simulink model "Gesamtsystem"  (R2018b)
settings: Solver=FixedStepDiscrete  StartTime=0.0  StopTime=1  RelTol=1e-3  EnableMultiTasking=on
libraries: c2833xlib x12, commutil2 x12, c280xlib x9, powerlib_extras x2, simulink x1, c2000lib x1, dspstat3 x1
(part 2 of 3)

== system Gesamtsystem/Subsystem/Subsystem2 ==
  In1 : Inport
  In2 : Inport  Port=2
  Drehrichtungsvorgabe für einen Motor1 : c2833xlib/Digital Output  GPIO_Number=GPIO16~GPIO23  GPIO_Bit0=on  GPIO_BIT0_Toggle=off  GPIO_Bit1=off  GPIO_BIT1_Toggle=off  GPIO_Bit2=off  GPIO_BIT2_Toggle=off  GPIO_Bit3=off  GPIO_BIT3_Toggle=off  GPIO_Bit4=off  GPIO_BIT4_Toggle=off  GPIO_Bit5=off  GPIO_BIT5_Toggle=off  GPIO_Bit6=off  GPIO_BIT6_Toggle=off  GPIO_Bit7=off  GPIO_BIT7_Toggle=off
      settings: SourceProductName=Embedded Coder Support Package for Texas Instruments C2000 Processors  SourceProductBaseCode=TIC2000
  PWM Vorgabe für einen Motor 1 : c280xlib/ePWM  checkMode=off  useModule=ePWM6  periodUnits=Clock cycles  timerSource=Specify via dialog  timerPeriod_clk=64000  timerPeriod_sec=0.0001  tbshadow=Counter equals to zero  countingMode=Up  phaseActiveEnable=Disable  phaseDirection=Count down after sync  phaseActive=0  synchronizationEnable=off  synchronizationOption=Disable  clockPrescale=1  HSclockPrescale=1  ePWMxAStatus=off  CMPAUnits=Clock cycles  CMPASource=Specify via dialog  CMPAValue_per=50  CMPAValue_clk=32000  enCMPAshadow=Counter equals to zero  ePWMxAactionLogic1=Do nothing  ePWMxAactionLogic2=Clear  ePWMxAactionLogic3=Set  ePWMxAactionLogic4=Do nothing  ePWMxAactionLogic5=Do nothing  ePWMxAactionLogic6=Do nothing  ePWMxALoadMode=Load on counter equals to zero (CTR=Zero)  ePWMxACSFenable=off  ePWMxACSFvalue=Forcing disable  ePWMxASFreload=Zero  enHRPWM=off  HRPWM_LoadMode=Counter equals to zero (CTR=ZERO)  HRPWM_CTLMode=Phase control mode  HRPWM_EDGMode=Both edge  enSFO=on  ePWMxBStatus=on  CMPBUnits=Percentages  CMPBSource=Input port  CMPBValue_per=0  CMPBValue_clk=32000  enCMPBshadow=Counter equals to zero  ePWMxBactionLogic1=Do nothing  ePWMxBactionLogic2=Set  ePWMxBactionLogic3=Do nothing  ePWMxBactionLogic4=Do nothing  ePWMxBactionLogic5=Clear  ePWMxBactionLogic6=Do nothing  ePWMxBLoadMode=Load on counter equals to zero (CTR=Zero)  ePWMxBCSFenable=off  ePWMxBCSFvalue=Forcing disable  ePWMxBSFreload=Zero  enableDBePWMxA=off  enableDBePWMxB=off  DBpolarity=Active high (AH)  DBedgeDelay=Positive  DBSource_ePWMxA=ePWMxA  DBSource_ePWMxB=ePWMxA  DBperiodSource=Specify via dialog  REDperiod=0  FEDperiod=0  adcstartModuleA=off  adcrequestEventA=First event  adcstartEventA=Counter equals to zero (CTR=Zero)  adcstartModuleB=off  adcrequestEventB=First event  adcstartEventB=Counter equals to zero (CTR=Zero)  intEn=off  intPrd=First event  intSel=Counter equals to zero (CTR=Zero)  chopperEnable=off  chopperFrequency=1  chopperFirstwidth=1  chopperDuty=12.5%  tripZonesource=Specify via dialog  tzselOSHT1=off  tzselOSHT2=off  tzselOSHT3=off  tzselOSHT4=off  tzselOSHT5=off  tzselOSHT6=off  tzselCBC1=off  tzselCBC2=off  tzselCBC3=off  tzselCBC4=off  tzselCBC5=off  tzselCBC6=off  enTzOstIntr=off  enTzCbcIntr=off  ePWMxAforced=No action  ePWMxBforced=No action  timerPeriod=-1  ePWMxAValue=0  ePWMxBValue=0  tripZoneoption=One-shot trip (OSHT)
      settings: SourceProductName=Embedded Coder Support Package for Texas Instruments C2000 Processors  SourceProductBaseCode=TIC2000
  wires:
  In2/1 -> Drehrichtungsvorgabe für einen Motor1/1
  In1/1 -> PWM Vorgabe für einen Motor 1/1

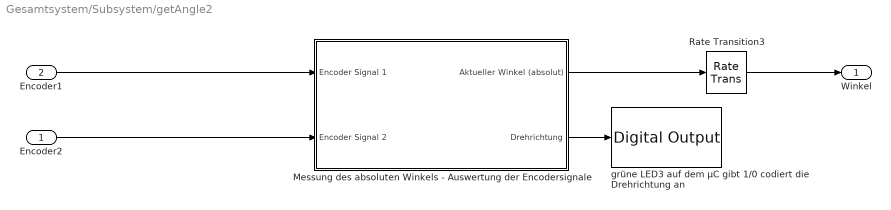
== system Gesamtsystem/Subsystem/getAngle2 ==
  Encoder2 : Inport
  Encoder1 : Inport  Port=2
  Messung des absoluten Winkels - Auswertung der Encodersignale : Subsystem
  Rate Transition3 : RateTransition  OutPortSampleTime=0.01
  grüne LED3 auf dem µC gibt 1/0 codiert die Drehrichtung an : c2833xlib/Digital Output  GPIO_Number=GPIO32~GPIO39  GPIO_Bit0=off  GPIO_BIT0_Toggle=off  GPIO_Bit1=off  GPIO_BIT1_Toggle=off  GPIO_Bit2=on  GPIO_BIT2_Toggle=off  GPIO_Bit3=off  GPIO_BIT3_Toggle=off  GPIO_Bit4=off  GPIO_BIT4_Toggle=off  GPIO_Bit5=off  GPIO_BIT5_Toggle=off  GPIO_Bit6=off  GPIO_BIT6_Toggle=off  GPIO_Bit7=off  GPIO_BIT7_Toggle=off
      settings: SourceProductName=Embedded Coder Support Package for Texas Instruments C2000 Processors  SourceProductBaseCode=TIC2000
  Winkel : Outport
  wires:
  Encoder1/1 -> Messung des absoluten Winkels - Auswertung der Encodersignale/1(Encoder Signal 1)
  Messung des absoluten Winkels - Auswertung der Encodersignale/2(Drehrichtung) -> grüne LED3 auf dem µC gibt 1/0 codiert die Drehrichtung an/1
  Messung des absoluten Winkels - Auswertung der Encodersignale/1(Aktueller Winkel (absolut)) -> Rate Transition3/1
  Encoder2/1 -> Messung des absoluten Winkels - Auswertung der Encodersignale/2(Encoder Signal 2)
  Rate Transition3/1 -> Winkel/1

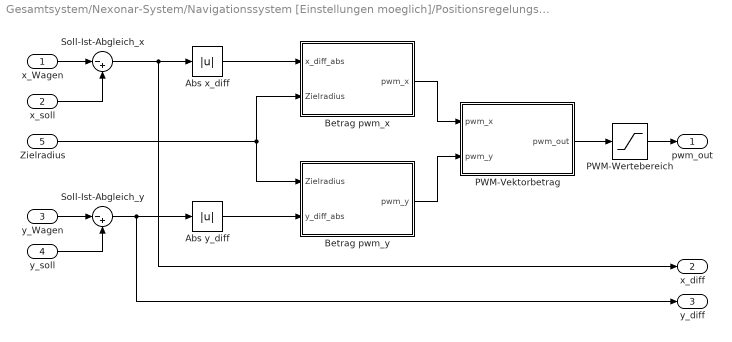
== system Gesamtsystem/Nexonar-System/Navigationssystem [Einstellungen moeglich]/Positionsregelungssystem (Soll-Ist-Abgleich & PWM-Auswertung) ==
  x_Wagen : Inport
  x_soll : Inport  Port=2
  y_Wagen : Inport  Port=3
  y_soll : Inport  Port=4
  Zielradius : Inport  Port=5
  Abs x_diff : Abs  SampleTime=0.01
  Abs y_diff : Abs  SampleTime=0.01
  Betrag pwm_x : MATLAB Function  TreatAsAtomicUnit=on  SystemSampleTime=0.01
  Betrag pwm_y : MATLAB Function  TreatAsAtomicUnit=on  SystemSampleTime=0.01
  PWM-Vektorbetrag : MATLAB Function  TreatAsAtomicUnit=on
  PWM-Wertebereich : Saturate  UpperLimit=100  LowerLimit=0
  Soll-Ist-Abgleich_x : Sum  Inputs=|-+  SampleTime=0.01
  Soll-Ist-Abgleich_y : Sum  Inputs=|-+  AccumDataTypeStr=double  SampleTime=0.01
  pwm_out : Outport
  x_diff : Outport  Port=2
  y_diff : Outport  Port=3
  wires:
  Soll-Ist-Abgleich_x/1 -> x_diff/1, Abs x_diff/1
  Abs x_diff/1 -> Betrag pwm_x/1(x_diff_abs)
  x_soll/1 -> Soll-Ist-Abgleich_x/2
  x_Wagen/1 -> Soll-Ist-Abgleich_x/1
  y_Wagen/1 -> Soll-Ist-Abgleich_y/1
  y_soll/1 -> Soll-Ist-Abgleich_y/2
  Soll-Ist-Abgleich_y/1 -> Abs y_diff/1, y_diff/1
  Abs y_diff/1 -> Betrag pwm_y/2(y_diff_abs)
  PWM-Wertebereich/1 -> pwm_out/1
  PWM-Vektorbetrag/1(pwm_out) -> PWM-Wertebereich/1
  Betrag pwm_x/1(pwm_x) -> PWM-Vektorbetrag/1(pwm_x)
  Betrag pwm_y/1(pwm_y) -> PWM-Vektorbetrag/2(pwm_y)
  Zielradius/1 -> Betrag pwm_y/1(Zielradius), Betrag pwm_x/2(Zielradius)

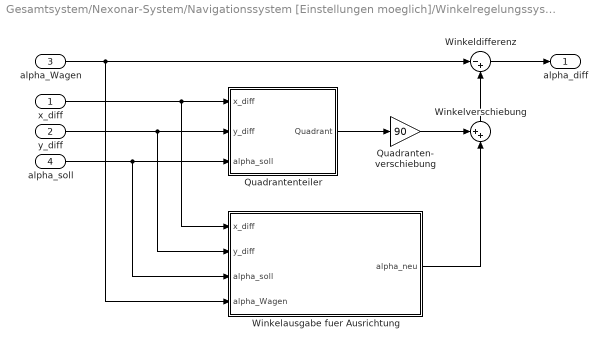
== system Gesamtsystem/Nexonar-System/Navigationssystem [Einstellungen moeglich]/Winkelregelungssystem (Soll-Ist-Abgleich & Ausrichtungsauswertung) ==
  x_diff : Inport
  y_diff : Inport  Port=2
  alpha_Wagen : Inport  Port=3
  alpha_soll : Inport  Port=4
  Quadranten- verschiebung : Gain  Gain=90
  Quadrantenteiler : Stateflow chart  TreatAsAtomicUnit=on
  Winkelausgabe fuer Ausrichtung : Stateflow chart  TreatAsAtomicUnit=on
  Winkeldifferenz : Sum  Inputs=|-+
  Winkelverschiebung : Sum  Inputs=++|
  alpha_diff : Outport
  wires:
  alpha_Wagen/1 -> Winkelausgabe fuer Ausrichtung/4(alpha_Wagen), Winkeldifferenz/1
  y_diff/1 -> Winkelausgabe fuer Ausrichtung/2(y_diff), Quadrantenteiler/2(y_diff)
  Winkelausgabe fuer Ausrichtung/1(alpha_neu) -> Winkelverschiebung/2
  Winkelverschiebung/1 -> Winkeldifferenz/2
  x_diff/1 -> Winkelausgabe fuer Ausrichtung/1(x_diff), Quadrantenteiler/1(x_diff)
  Quadrantenteiler/1(Quadrant) -> Quadranten- verschiebung/1
  Winkeldifferenz/1 -> alpha_diff/1
  Quadranten- verschiebung/1 -> Winkelverschiebung/1
  alpha_soll/1 -> Winkelausgabe fuer Ausrichtung/3(alpha_soll), Quadrantenteiler/3(alpha_soll)

== system Gesamtsystem/Nexonar-System/Nexonar-Positionsbestimmung/I2C Reset (behebt Stabilitätsprobleme der I2C-Verbindung) ==
  I2C Reinitialisierung : Subsystem  TreatAsAtomicUnit=on
  I2C Reset : Subsystem  TreatAsAtomicUnit=on
  Pulse Generator : DiscretePulseGenerator  Period=250  SampleTime=0.01
  wires:
  Pulse Generator/1 -> I2C Reinitialisierung/Trigger, I2C Reset/Trigger

== system Gesamtsystem/Nexonar-System/Nexonar-Positionsbestimmung/Triggered Subsystem ==
  Trigger : TriggerPort  TriggerType=function-call  VariantControl=(inherit)
  Delay : Delay  DelayLength=1  InitialCondition=0
  I2C Receive : c280xlib/I2C Receive  selectModule=I2C_A  addrFormat=7-Bit addressing  saSource=Specify via dialog  SAR=80  bitCount=8  dataLength=10  initValue=0  NACK=on  STP=off  STR=on  sampleTime=-1  dataType=uint8
      settings: SourceProductName=Embedded Coder Support Package for Texas Instruments C2000 Processors  SourceProductBaseCode=TIC2000
  Terminator : Terminator
  Vector Concatenate : Concatenate
  I2C_Read_Data : Outport
  wires:
  I2C Receive/2 -> Terminator/1
  I2C Receive/1 -> Vector Concatenate/2, Delay/1
  Delay/1 -> Vector Concatenate/1
  Vector Concatenate/1 -> I2C_Read_Data/1

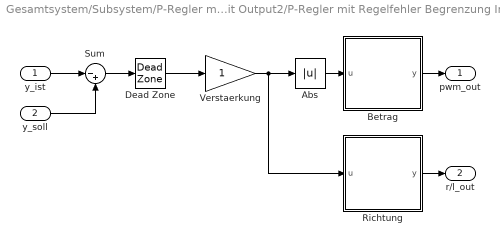
== system Gesamtsystem/Subsystem/P-Regler mit Output2/P-Regler mit Regelfehler Begrenzung Initial: k = 0.1, limiit = +//- 100 Sampletime 0.01 ==
  y_ist : Inport
  y_soll : Inport  Port=2
  Abs : Abs  SampleTime=0.01
  Betrag : MATLAB Function  TreatAsAtomicUnit=on  SystemSampleTime=0.01
  Dead Zone : DeadZone  SampleTime=0.01  SaturateOnIntegerOverflow=on
  Richtung : MATLAB Function  TreatAsAtomicUnit=on  SystemSampleTime=0.01
  Sum : Sum  Inputs=|-+  SampleTime=0.01
  Verstaerkung : Gain  SampleTime=0.01
  pwm_out : Outport
  r/l_out : Outport  Port=2
  wires:
  Betrag/1(y) -> pwm_out/1
  Sum/1 -> Dead Zone/1
  Verstaerkung/1 -> Abs/1, Richtung/1(u)
  Dead Zone/1 -> Verstaerkung/1
  Abs/1 -> Betrag/1(u)
  y_soll/1 -> Sum/2
  Richtung/1(y) -> r/l_out/1
  y_ist/1 -> Sum/1

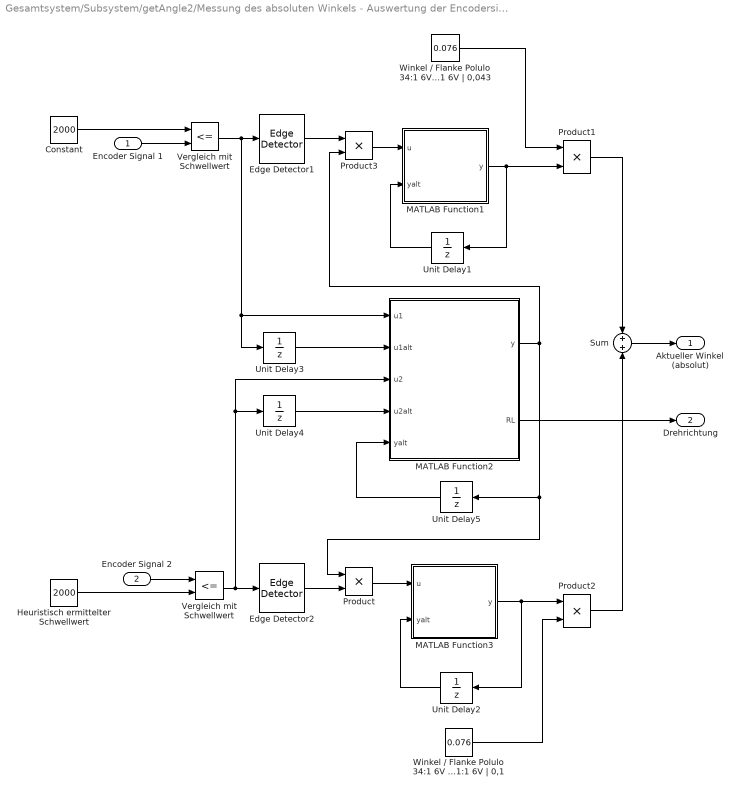
== system Gesamtsystem/Subsystem/getAngle2/Messung des absoluten Winkels - Auswertung der Encodersignale ==
  Encoder Signal 1 : Inport
  Encoder Signal 2 : Inport  Port=2
  Constant : Constant  Value=2000
  Edge Detector1 : powerlib_extras/Control  Blocks/Edge Detector  model=Either  ic=0
  Edge Detector2 : powerlib_extras/Control  Blocks/Edge Detector  model=Either  ic=0
  Heuristisch ermittelter Schwellwert : Constant  Value=2000
  MATLAB Function1 : MATLAB Function  TreatAsAtomicUnit=on
  MATLAB Function2 : MATLAB Function  TreatAsAtomicUnit=on
  MATLAB Function3 : MATLAB Function  TreatAsAtomicUnit=on
  Product{,1..3} (4 alike) : Product  RndMeth=Zero
  Sum : Sum  Inputs=+|+
  Unit Delay{1..5} (5 alike) : UnitDelay  SampleTime=-1
  Vergleich mit Schwellwert : RelationalOperator  Operator=<=  OutDataTypeStr=boolean  RndMeth=Nearest
  Vergleich mit Schwellwert : RelationalOperator  Operator=<=  OutDataTypeStr=boolean  RndMeth=Nearest
  Winkel / Flanke Polulo 34:1 6V | 0,22 Polulo 74:1 6V | 0,1 Polulo 98:1 6V | 0,076 Polulo 171:1 6V | 0,043 : Constant  Value=0.076
  Winkel / Flanke Polulo 34:1 6V | 0,22 Polulo 74:1 6V | 0,1 Polulo 98:1 6V | 0,076 Polulo 171:1 6V | 0,1 : Constant  Value=0.076
  Aktueller Winkel (absolut) : Outport
  Drehrichtung : Outport  Port=2
  wires:
  Vergleich mit Schwellwert/1 -> Unit Delay4/1, MATLAB Function2/3(u2), Edge Detector2/1
  Sum/1 -> Aktueller Winkel (absolut)/1
  Vergleich mit Schwellwert/1 -> Edge Detector1/1, Unit Delay3/1, MATLAB Function2/1(u1)
  Heuristisch ermittelter Schwellwert/1 -> Vergleich mit Schwellwert/2
  Unit Delay2/1 -> MATLAB Function3/2(yalt)
  Encoder Signal 1/1 -> Vergleich mit Schwellwert/2
  MATLAB Function3/1(y) -> Unit Delay2/1, Product2/1
  Product1/1 -> Sum/1
  Constant/1 -> Vergleich mit Schwellwert/1
  Encoder Signal 2/1 -> Vergleich mit Schwellwert/1
  Product2/1 -> Sum/2
  Unit Delay1/1 -> MATLAB Function1/2(yalt)
  MATLAB Function1/1(y) -> Product1/2, Unit Delay1/1
  Winkel / Flanke Polulo 34:1 6V | 0,22 Polulo 74:1 6V | 0,1 Polulo 98:1 6V | 0,076 Polulo 171:1 6V | 0,043/1 -> Product1/1
  Product3/1 -> MATLAB Function1/1(u)
  Product/1 -> MATLAB Function3/1(u)
  Edge Detector1/1 -> Product3/1
  Unit Delay3/1 -> MATLAB Function2/2(u1alt)
  Unit Delay4/1 -> MATLAB Function2/4(u2alt)
  Edge Detector2/1 -> Product/2
  MATLAB Function2/1(y) -> Product/1, Unit Delay5/1, Product3/2
  Winkel / Flanke Polulo 34:1 6V | 0,22 Polulo 74:1 6V | 0,1 Polulo 98:1 6V | 0,076 Polulo 171:1 6V | 0,1/1 -> Product2/2
  MATLAB Function2/2(RL) -> Drehrichtung/1
  Unit Delay5/1 -> MATLAB Function2/5(yalt)

== system Gesamtsystem/Nexonar-System/Nexonar-Positionsbestimmung/I2C Reset (behebt Stabilitätsprobleme der I2C-Verbindung)/I2C Reinitialisierung ==
  Trigger : TriggerPort  TriggerType=falling  VariantControl=(inherit)
  I2C Reinitialisierung : MATLAB Function  TreatAsAtomicUnit=on

== system Gesamtsystem/Nexonar-System/Nexonar-Positionsbestimmung/I2C Reset (behebt Stabilitätsprobleme der I2C-Verbindung)/I2C Reset ==
  Trigger : TriggerPort  VariantControl=(inherit)
  I2C Reset : MATLAB Function  TreatAsAtomicUnit=on

== stateflow chart Gesamtsystem/Nexonar-System/Nexonar-Positionsbestimmung/Chart1 ==
  state Daten_einlesen
  state x0
  state x1_1
    entry: int16z_bin[0] = int8z_1[0];
    int16z_bin[1] = int8z_1[1];
    int16z_bin[2] = int8z_1[2];
    int16z_bin[3] = int8z_1[3];
    int16z_bin[4] = int8z_1[4];
    int16z_bin[5] = int8z_1[5]
    int16z_bin[6] = int8z_1[6];
    int16z_bin[7] = int8z_1[7];
    int16z_bin[8] = int8z_2[0];
    int16z_bin[9] = int8z_2[1];
    int16z_bin[10] = int8z_2[2];
    int16z_bin[11] = int8z_2[3];
    int16z_bin[12] = int8z_2[4];
    int16z_bin[13] = int8z_2[5]
    int16z_bin[14] = int8z_2[6];
    int16z_bin[15] = int8z_2[7];
  x0 -> Daten_einlesen
  (default) -> x0
  Daten_einlesen -> x1_1
  x1_1 -> Daten_einlesen
  data: int8z_1 input size=8; int8z_2 input size=8; int16z_bin output size=16 =0

== matlab function Gesamtsystem/Nexonar-System/Navigationssystem [Einstellungen moeglich]/Positionsregelungssystem (Soll-Ist-Abgleich & PWM-Auswertung)/PWM-Vektorbetrag ==
  data: pwm_x input; pwm_out output; pwm_y input
function pwm_out = fcn(pwm_x, pwm_y)

pwm_out = round(sqrt(pwm_x * pwm_x + pwm_y * pwm_y));

== stateflow chart Gesamtsystem/Add-Ons-Ansteuerung [Einstellungen moeglich] Achtung! Einige Einstellungswerte haengen von den Werten im Nexonar-System ab./Beendigung-System [Einstellungen moeglich]/Beendigung-Ansteuerung ==
  state Start_Warten
  state Aus_Zustand
    entry:
    aus_an = 0;
  state Anschalten
    entry:
    aus_an = 1;
  (default) -> Start_Warten
  Start_Warten -> Aus_Zustand
  Aus_Zustand -> Anschalten [order 1] : [Shutdown == 1]
  Aus_Zustand -> Anschalten [order 2] : [Fahrzeug_Motoren(1) == 0 && Fahrzeug_Motoren(2) == 0 ...
      | && Fahrzeug_Motoren(3) == Fahrzeug_Motoren(4)]
  data: aus_an output; Fahrzeug_Motoren input; Shutdown input

== matlab function Gesamtsystem/Nexonar-System/Konvertierung Nexonar -> Fahrzeug Folgende Werte koennen für Nexonar eingestellt werden: - r_Versatz_Nexo: Radialer Versatz des Nexonars zur Rotationsachse des Fahrzeugs - phi_Versatz_Nexo: Winkelversatz des Nexonars gegenüber der x-Achse (Mittelpunkt: Rotationspunkt des Fahrzeugs) - psi_Offset_Nexo: Winkelversatz des Nexonars gegenüber der x-Achse (Mittelpunkt: Nexonar-Empfangstelle) ==
  data: x_ist input; x_Wagen output; y_ist input; alpha_ist input; y_Wagen output; alpha_Wagen output
function [x_Wagen, y_Wagen, alpha_Wagen] = fcn(x_ist, y_ist, alpha_ist)

r_Versatz_Nexo = 2.5; % in mm
phi_Versatz_Nexo = 30; % in °
psi_Offset_Nexo = 15; % in 


alpha_Wagen = alpha_ist - psi_Offset_Nexo;
x_Wagen = x_ist - round(r_Versatz_Nexo * cos((phi_Versatz_Nexo+alpha_Wagen)*2*pi/360));
y_Wagen = y_ist - round(r_Versatz_Nexo * sin((phi_Versatz_Nexo+alpha_Wagen)*2*pi/360));

== stateflow chart Gesamtsystem/Nexonar-System/Fahrablaufsteuerung [Init: Zielradius = 10mm] Gang = 0: vorwaerts Gang = 1: rueckwaerts Folgende Werte fuer den Ablauf sind einstellbar: - Zielkoordinatenwerte - Gangwert ==
  state Parken
    state Parken_1
      entry:
      x_soll = 1420;
      y_soll = -50;
      alpha_soll = -1;
    state Wechsel_1
      entry:
      Counter = Counter + 1;
    state Parken_2
      entry:
      x_soll = 1620;
      y_soll = -135;
      alpha_soll = -1;
    state Wechsel_2
      entry:
      Counter = Counter + 1;
    state Parken_3
      entry:
      x_soll = 1640;
      y_soll = -131;
      alpha_soll = -1;
    state Wechsel_3
      entry:
      Counter = Counter + 1;
    (default) -> Parken_1 : {Counter = 0}
    Parken_1 -> Parken.Wechsel_1 : [abs(x_soll - x_Wagen) <= Zielradius && abs(y_soll - y_Wagen) <= Zielradius]
    Parken.Wechsel_1 -> Parken_2
    Parken_2 -> Parken.Wechsel_2 : [abs(x_soll - x_Wagen) <= Zielradius && abs(y_soll - y_Wagen) <= Zielradius]
    Parken.Wechsel_2 -> Parken_3
    Parken_3 -> Parken.Wechsel_3 : [abs(x_soll - x_Wagen) <= Zielradius && abs(y_soll - y_Wagen) <= Zielradius]
  state Uebergabe
    state Uebergabepunkt_x_Richtung
      entry:
      x_soll = x_least;
      y_soll = y_least;
      alpha_soll = -1;
    state Wechsel_1
      entry:
      Counter = Counter + 1;
    state Uebergabepunkt_y_Richtung
      entry:
      x_soll = x_least;
      y_soll = 50;
      alpha_soll = 80;
    state Warten_Uebergabe
    state Wechsel_2
      entry:
      Counter = Counter + 1;
    (default) -> Uebergabepunkt_x_Richtung : {Counter = 0}
    Uebergabepunkt_x_Richtung -> Uebergabe.Wechsel_1 : [abs(x_soll - x_Wagen) <= Zielradius && abs(y_soll - y_Wagen) <= Zielradius]
        | {x_least = x_soll; y_least = y_soll;}
    Uebergabe.Wechsel_1 -> Uebergabepunkt_y_Richtung
    Uebergabepunkt_y_Richtung -> Warten_Uebergabe [order 1] : [Uebergabe == 1]
    Uebergabepunkt_y_Richtung -> Warten_Uebergabe [order 2] : [abs(x_soll - x_Wagen) <= Zielradius && abs(y_soll - y_Wagen) <= Zielradius]
    Warten_Uebergabe -> Uebergabe.Wechsel_2 : [after(10,sec)]
  state Start_Einstellung_Init
    entry:
    Zielradius = 10;
  state Sammeln
    state Anfahrpunkt_1
      entry:
      x_soll = 1500;
      y_soll = 0;
      alpha_soll = -1;
    state Wechsel_1
      entry:
      Counter = Counter + 1;
    state Anfahrpunkt_2
      entry:
      x_soll = 1200;
      y_soll = 100;
      alpha_soll = -1;
    state Wechsel_2
      entry:
      Counter = Counter + 1;
    state Anfahrpunkt_3
      entry:
      x_soll = 1000;
      y_soll = 250;
      alpha_soll = -1;
    state Wechsel_3
      entry:
      Counter = Counter + 1;
    state Anfahrpunkt_4
      entry:
      x_soll = 940;
      y_soll = 650;
      alpha_soll = -1;
    state Wechsel_4
      entry:
      Counter = Counter + 1;
    state Anfahrpunkt_5
      entry:
      x_soll = 850;
      y_soll = 750;
      alpha_soll = -1;
    state Wechsel_5
      entry:
      Counter = Counter + 1;
    state Anfahrpunkt_6
      entry:
      x_soll = 600;
      y_soll = 825;
      alpha_soll = -1;
    state Wechsel_6
      entry:
      Counter = Counter + 1;
    state Wechsel_10
      entry:
      Counter = Counter + 1;
    state Anfahrpunkt_7
      entry:
      x_soll = 500;
      y_soll = 825;
      alpha_soll = -1;
    state Anfahrpunkt_10
      entry:
      x_soll = 880;
      y_soll = 0;
      alpha_soll = -1;
    state Wechsel_7
      entry:
      Counter = Counter + 1;
    state Anfahrpunkt_8
      entry:
      x_soll = 325;
      y_soll = 725;
      alpha_soll = -1;
    state Wechsel_8
      entry:
      Counter = Counter + 1;
    state Anfahrpunkt_9
      entry:
      x_soll = 400;
      y_soll = 300;
      alpha_soll = -1;
    state Wechsel_9
      entry:
      Counter = Counter + 1;
    state Anfahrpunkt_11
      entry:
      x_soll = 600;
      y_soll = 0;
      alpha_soll = -1;
    state Wechsel_11
      entry:
      Counter = Counter + 1;
    state Anfahrpunkt_12
      entry:
      x_soll = 900;
      y_soll = 0;
      alpha_soll = -1;
    state Wechsel_12
      entry:
      Counter = Counter + 1;
    state Anfahrpunkt_13
      entry:
      x_soll = 1200;
      y_soll = 0;
      alpha_soll = -1;
    state Wechsel_13
      entry:
      Counter = Counter + 1;
    state Anfahrpunkt_14
      entry:
      x_soll = 1370;
      y_soll = -100;
      alpha_soll = -1;
    state Wechsel_14
      entry:
      Counter = Counter + 1;
    (default) -> Anfahrpunkt_1 : {Counter = 0}
    Anfahrpunkt_1 -> Sammeln.Wechsel_1 : [abs(x_soll - x_Wagen) <= Zielradius && abs(y_soll - y_Wagen) <= Zielradius]
    Sammeln.Wechsel_1 -> Anfahrpunkt_2
    Anfahrpunkt_2 -> Sammeln.Wechsel_2 : [abs(x_soll - x_Wagen) <= Zielradius && abs(y_soll - y_Wagen) <= Zielradius]
    Sammeln.Wechsel_2 -> Anfahrpunkt_3
    Anfahrpunkt_3 -> Sammeln.Wechsel_3 : [abs(x_soll - x_Wagen) <= Zielradius && abs(y_soll - y_Wagen) <= Zielradius]
    Sammeln.Wechsel_3 -> Anfahrpunkt_4
    Wechsel_10 -> Anfahrpunkt_4
    Anfahrpunkt_4 -> Wechsel_4 : [abs(x_soll - x_Wagen) <= Zielradius && abs(y_soll - y_Wagen) <= Zielradius]
    Wechsel_4 -> Anfahrpunkt_5
    Anfahrpunkt_5 -> Wechsel_5 : [abs(x_soll - x_Wagen) <= Zielradius && abs(y_soll - y_Wagen) <= Zielradius]
    Wechsel_5 -> Anfahrpunkt_6
    Anfahrpunkt_6 -> Wechsel_6 : [abs(x_soll - x_Wagen) <= Zielradius && abs(y_soll - y_Wagen) <= Zielradius]
    Wechsel_6 -> Anfahrpunkt_7
    Anfahrpunkt_10 -> Wechsel_10 : [abs(x_soll - x_Wagen) <= Zielradius && abs(y_soll - y_Wagen) <= Zielradius]
    Anfahrpunkt_7 -> Wechsel_7 : [abs(x_soll - x_Wagen) <= Zielradius && abs(y_soll - y_Wagen) <= Zielradius]
    Wechsel_9 -> Anfahrpunkt_10 [order 1] : [Counter == 9]
    Wechsel_7 -> Anfahrpunkt_8
    Anfahrpunkt_8 -> Wechsel_8 : [abs(x_soll - x_Wagen) <= Zielradius && abs(y_soll - y_Wagen) <= Zielradius]
    Wechsel_8 -> Anfahrpunkt_9
    Anfahrpunkt_9 -> Wechsel_9 : [abs(x_soll - x_Wagen) <= Zielradius && abs(y_soll - y_Wagen) <= Zielradius]
    Wechsel_9 -> Anfahrpunkt_11 [order 2]
    Anfahrpunkt_11 -> Wechsel_11 : [abs(x_soll - x_Wagen) <= Zielradius && abs(y_soll - y_Wagen) <= Zielradius]
    Wechsel_11 -> Anfahrpunkt_12
    Anfahrpunkt_12 -> Wechsel_12 : [abs(x_soll - x_Wagen) <= Zielradius && abs(y_soll - y_Wagen) <= Zielradius]
    Wechsel_12 -> Anfahrpunkt_13
    Anfahrpunkt_13 -> Wechsel_13 : [abs(x_soll - x_Wagen) <= Zielradius && abs(y_soll - y_Wagen) <= Zielradius]
    Wechsel_13 -> Anfahrpunkt_14
    Anfahrpunkt_14 -> Wechsel_14 : [abs(x_soll - x_Wagen) <= Zielradius && abs(y_soll - y_Wagen) <= Zielradius]
  state Ende
  (default) -> Start_Einstellung_Init
  Start_Einstellung_Init -> Sammeln : {Gang = 0;
      | alpha_soll = -1;}
  Uebergabe -> Parken : [Counter == 2]{Gang = 0}
  Sammeln -> Uebergabe : [Counter == 20]
      | {Gang = 1;
      | x_least = x_soll;
      | y_least = y_soll;}
  Parken -> Ende : [Counter == 3]
  data: x_soll output; y_soll output; alpha_soll output; x_Wagen input; y_Wagen input; Counter local; x_least local; y_least local; Gang output; Zielradius output; Uebergabe input

== stateflow chart Gesamtsystem/Add-Ons-Ansteuerung [Einstellungen moeglich] Achtung! Einige Einstellungswerte haengen von den Werten im Nexonar-System ab./Zylindermotor-System [Einstellungen moeglich] Achtung! Einige Einstellungswerte haengen von den Werten im Nexonar-System ab./Zylindermotor-Ansteuerung Folgende Werte sind einstellbar: - Drehstaerke (in %) (-> ZM_pwm_out in "Ausfuerung") - Drehrichtung (rechts = 0, links = 1) (-> ZM_r_l_out in "Init_und_Warten") - Drehdauer (-> zwischen "Ausfuehrung" und "Beendet") - Ausfuehrungspunkt (in mm) [durch Wechsel der Soll-Position] (-> zwischen "Init_und_Start" und "Ausfuehrung) Wichtig! Der Ausfuerungspunkt haengt von den EXAKTEN Soll-Werten aus der Fahrablaufsteuerung im Nexonar-System ab. ==
  state Init_und_Warten
    entry:
    ZM_pwm_out = 0;
    ZM_r_l_out = 1;
  state Ausfuehrung
    entry:
    ZM_pwm_out = 50;
  state Beendet
    entry:
    ZM_pwm_out = 0;
  Init_und_Warten -> Ausfuehrung : [x_soll == 1200 && y_soll == 0]
  (default) -> Init_und_Warten
  Ausfuehrung -> Beendet : [after(0.1,sec)]
  data: ZM_pwm_out output; ZM_r_l_out output; x_soll input; y_soll input

== stateflow chart Gesamtsystem/Nexonar-System/Navigationssystem [Einstellungen moeglich]/Fahrsystem ==
  state Fahren_mit_Ausrichtungsregelung
    entry:
    pwm_out_l = pwm_out - round(pwm_mindern(1) * (pwm_out / 100) ^ 2) * l_mindern;
    pwm_out_r = pwm_out - round(pwm_mindern(1) * (pwm_out / 100) ^ 2) * r_mindern;
    r_l_out_l = 1 - Gang;
    r_l_out_r = 1 - Gang;
  state Start_Warten
  state Drehen_links_max
    entry:
    pwm_out_l = 100;
    pwm_out_r = 100;
    r_l_out_l = 0;
    r_l_out_r = 1;
  state Drehen_rechts_max
    entry:
    pwm_out_l = 100;
    pwm_out_r = 100;
    r_l_out_l = 1;
    r_l_out_r = 0;
  state Drehen_links_gesteuert
    entry:
    pwm_out_l = 59 + abs(alpha_diff_opt);
    pwm_out_r = 59 + abs(alpha_diff_opt);
    r_l_out_l = 0;
    r_l_out_r = 1;
  state Drehen_rechts_gesteuert
    entry:
    pwm_out_l = 59 + abs(alpha_diff_opt);
    pwm_out_r = 59 + abs(alpha_diff_opt);
    r_l_out_l = 1;
    r_l_out_r = 0;
  (junction 81) -> Fahren_mit_Ausrichtungsregelung [order 1] : [pwm_mindern(2) == 1]
      | {l_mindern = 1 - Gang; r_mindern = 0 + Gang;}
  (junction 81) -> Fahren_mit_Ausrichtungsregelung [order 2] : [pwm_mindern(2) == 0]
      | {l_mindern = 0 + Gang; r_mindern = 1 - Gang;}
  (junction 1) -> (junction 81) [order 2]
  Fahren_mit_Ausrichtungsregelung -> (junction 32)
  (junction 81) -> Fahren_mit_Ausrichtungsregelung [order 3] : {l_mindern = 0; r_mindern = 0;}
  Start_Warten -> (junction 1)
  (junction 32) -> (junction 1)
  (default) -> Start_Warten
  Drehen_links_max -> (junction 32)
  Drehen_rechts_max -> (junction 32)
  Drehen_links_gesteuert -> (junction 32)
  (junction 1) -> (junction 18) [order 1] : [abs(alpha_diff_opt) > 0 && pwm_out > 0]
  Drehen_rechts_gesteuert -> (junction 32)
  (junction 18) -> (junction 44) [order 1] : [abs(alpha_diff_opt) > 40]
  (junction 44) -> Drehen_links_max [order 1] : [alpha_diff_opt > 0]
  (junction 18) -> (junction 52) [order 2]
  (junction 44) -> Drehen_rechts_max [order 2]
  (junction 52) -> Drehen_links_gesteuert [order 1] : [alpha_diff_opt > 0]
  (junction 52) -> Drehen_rechts_gesteuert [order 2]
  data: Gang input; pwm_out input; pwm_mindern input; alpha_diff_opt input; pwm_out_l output; pwm_out_r output; r_l_out_l output; r_l_out_r output; l_mindern local; r_mindern local

== stateflow chart Gesamtsystem/Nexonar-System/Navigationssystem [Einstellungen moeglich]/Drehweg-Optimierung mit Gang-Ausrichtung [Init: Stillstandintervall = ±15°] ==
  state Einstellung_Init
    entry:
    Stillstandintervall = 15;
    %%%
    pwm_mindern = [0 0];
  state Drehstillstand_mit_Ausrichtungsregelung
    entry:
    alpha_diff_opt = 0;
    if abs(alpha_diff_intern) < 5
    pwm_mindern(1) = round(abs(alpha_diff_intern));
    elseif abs(alpha_diff_intern) < 15
    pwm_mindern(1) = 5 + floor((abs(alpha_diff_intern) - 5) / 2);
    else
    pwm_mindern(1) = 10;
    end;
    if alpha_diff_intern < 0
    pwm_mindern(2) = 0;
    elseif alpha_diff_intern > 0
    pwm_mindern(2) = 1;
    else
    pwm_mindern(2) = 2;
    end;
  state Weiterleitung_bei_Drehzustand
    entry:
    alpha_diff_opt = alpha_diff_intern;
  (default) -> Einstellung_Init
  (junction 95) -> (junction 32)
  Einstellung_Init -> (junction 32)
  (junction 32) -> (junction 6) : {alpha_diff_intern = alpha_diff + 180 * Gang}
  (junction 6) -> (junction 68) [order 2]
  (junction 68) -> Drehstillstand_mit_Ausrichtungsregelung [order 1] : [abs(alpha_diff_intern) <= Stillstandintervall]
  Drehstillstand_mit_Ausrichtungsregelung -> (junction 95)
  (junction 6) -> (junction 13) [order 1] : [abs(alpha_diff_intern) > 180]
  (junction 13) -> (junction 68) [order 1] : [alpha_diff_intern > 0]
      | {alpha_diff_intern = -360 + alpha_diff_intern}
  Weiterleitung_bei_Drehzustand -> (junction 95)
  (junction 13) -> (junction 68) [order 2] : {alpha_diff_intern = 360 + alpha_diff_intern}
  (junction 68) -> Weiterleitung_bei_Drehzustand [order 2]
  data: pwm_mindern output; Gang input; alpha_diff input; alpha_diff_opt output; alpha_diff_intern local; Stillstandintervall local

== stateflow chart Gesamtsystem/Nexonar-System/Motorsteuerung bei der Uebergabe ==
  state Start
  state Warten1
    entry:
    Value = 1;
  state Stehen
    entry:
    Value = 0;
  state Weiter
    entry:
    Value = 1;
  (default) -> Start
  Start -> Warten1 : [Uebergabe == 1]
  Stehen -> Weiter : [after(10,sec)]
  Warten1 -> Stehen : [Uebergabe == 1 && after(10,sec)]
  data: Uebergabe input; Value output

== stateflow chart Gesamtsystem/Nexonar-System/Navigationssystem [Einstellungen moeglich]/Winkelregelungssystem (Soll-Ist-Abgleich & Ausrichtungsauswertung)/Quadrantenteiler ==
  state Quadrant_a
    entry:
    Quadrant = 0;
  state Quadrant_b
    entry:
    Quadrant = 1;
  state Start_Warten
  state Quadrant_c
    entry:
    Quadrant = 2;
  state Quadrant_d
    entry:
    Quadrant = 3;
  (junction 6) -> Quadrant_a [order 1] : [alpha_soll ~= -1]
  Quadrant_a -> (junction 35)
  (junction 6) -> Quadrant_a [order 2] : [x_diff >= 0 && y_diff >= 0]
  (junction 6) -> Quadrant_b [order 3] : [x_diff <= 0 && y_diff > 0]
  Quadrant_b -> (junction 35)
  Start_Warten -> (junction 6)
  (junction 35) -> (junction 6)
  (default) -> Start_Warten
  (junction 6) -> Quadrant_c [order 4] : [x_diff < 0 && y_diff <= 0]
  Quadrant_c -> (junction 35)
  (junction 6) -> Quadrant_d [order 5]
  Quadrant_d -> (junction 35)
  data: x_diff input; y_diff input; Quadrant output; alpha_soll input

== stateflow chart Gesamtsystem/Nexonar-System/Navigationssystem [Einstellungen moeglich]/Winkelregelungssystem (Soll-Ist-Abgleich & Ausrichtungsauswertung)/Winkelausgabe fuer Ausrichtung ==
  state Ausrichtung_gegeben
    entry:
    alpha_neu = alpha_soll;
  state Ausrichtung_ohne_Aenderung
    entry:
    alpha_neu = alpha_Wagen;
  state Start_Warten
  state Trigonometrische_Auswertung_in_Grad_fuer_Quadrant_1_3
    entry:
    alpha_neu = round(atan(abs(x_diff)/abs(y_diff))*360/(2*pi));
  state Trigonometrische_Auswertung_in_Grad_fuer_Quadrant_0_2
    entry:
    alpha_neu = round(atan(abs(y_diff)/abs(x_diff))*360/(2*pi));
  Ausrichtung_gegeben -> (junction 65)
  (junction 4) -> Ausrichtung_gegeben [order 1] : [alpha_soll ~= -1]
  (junction 4) -> Ausrichtung_ohne_Aenderung [order 2] : [x_diff == 0 && y_diff == 0]
  Ausrichtung_ohne_Aenderung -> (junction 65)
  Start_Warten -> (junction 4)
  (junction 65) -> (junction 4)
  (default) -> Start_Warten
  (junction 4) -> Trigonometrische_Auswertung_in_Grad_fuer_Quadrant_1_3 [order 5]
  Trigonometrische_Auswertung_in_Grad_fuer_Quadrant_1_3 -> (junction 65)
  (junction 4) -> Trigonometrische_Auswertung_in_Grad_fuer_Quadrant_0_2 [order 3] : [x_diff > 0 && y_diff >= 0]
  (junction 4) -> Trigonometrische_Auswertung_in_Grad_fuer_Quadrant_0_2 [order 4] : [x_diff < 0 && y_diff <= 0]
  Trigonometrische_Auswertung_in_Grad_fuer_Quadrant_0_2 -> (junction 65)
  data: x_diff input; y_diff input; alpha_soll input; alpha_neu output; alpha_Wagen input

== stateflow chart Gesamtsystem/Nexonar-System/Nexonar-Positionsbestimmung/Chart2 ==
  state Daten_einlesen
  state x0
  state x1_1
    entry: int16y_bin[0] = int8y_1[0];
    int16y_bin[1] = int8y_1[1];
    int16y_bin[2] = int8y_1[2];
    int16y_bin[3] = int8y_1[3];
    int16y_bin[4] = int8y_1[4];
    int16y_bin[5] = int8y_1[5]
    int16y_bin[6] = int8y_1[6];
    int16y_bin[7] = int8y_1[7];
    int16y_bin[8] = int8y_2[0];
    int16y_bin[9] = int8y_2[1];
    int16y_bin[10] = int8y_2[2];
    int16y_bin[11] = int8y_2[3];
    int16y_bin[12] = int8y_2[4];
    int16y_bin[13] = int8y_2[5]
    int16y_bin[14] = int8y_2[6];
    int16y_bin[15] = int8y_2[7];
  x0 -> Daten_einlesen
  (default) -> x0
  Daten_einlesen -> x1_1
  x1_1 -> Daten_einlesen
  data: int8y_1 input size=8; int8y_2 input size=8; int16y_bin output size=16 =0

== stateflow chart Gesamtsystem/Nexonar-System/Nexonar-Positionsbestimmung/Chart4 ==
  state Daten_einlesen
  state x0
  state x1_1
    entry: int16a1_bin[0] = int8a1_1[0];
    int16a1_bin[1] = int8a1_1[1];
    int16a1_bin[2] = int8a1_1[2];
    int16a1_bin[3] = int8a1_1[3];
    int16a1_bin[4] = int8a1_1[4];
    int16a1_bin[5] = int8a1_1[5]
    int16a1_bin[6] = int8a1_1[6];
    int16a1_bin[7] = int8a1_1[7];
    int16a1_bin[8] = int8a1_2[0];
    int16a1_bin[9] = int8a1_2[1];
    int16a1_bin[10] = int8a1_2[2];
    int16a1_bin[11] = int8a1_2[3];
    int16a1_bin[12] = int8a1_2[4];
    int16a1_bin[13] = int8a1_2[5]
    int16a1_bin[14] = int8a1_2[6];
    int16a1_bin[15] = int8a1_2[7];
  x0 -> Daten_einlesen
  (default) -> x0
  Daten_einlesen -> x1_1
  x1_1 -> Daten_einlesen
  data: int8a1_1 input size=8; int8a1_2 input size=8; int16a1_bin output size=16 =0

== stateflow chart Gesamtsystem/Nexonar-System/Nexonar-Positionsbestimmung/Chart6 ==
  state Daten_einlesen
  state x0
  state x1_1
    entry: int16x_bin[0] = int8x_1[0];
    int16x_bin[1] = int8x_1[1];
    int16x_bin[2] = int8x_1[2];
    int16x_bin[3] = int8x_1[3];
    int16x_bin[4] = int8x_1[4];
    int16x_bin[5] = int8x_1[5]
    int16x_bin[6] = int8x_1[6];
    int16x_bin[7] = int8x_1[7];
    int16x_bin[8] = int8x_2[0];
    int16x_bin[9] = int8x_2[1];
    int16x_bin[10] = int8x_2[2];
    int16x_bin[11] = int8x_2[3];
    int16x_bin[12] = int8x_2[4];
    int16x_bin[13] = int8x_2[5]
    int16x_bin[14] = int8x_2[6];
    int16x_bin[15] = int8x_2[7];
  x0 -> Daten_einlesen
  (default) -> x0
  Daten_einlesen -> x1_1
  x1_1 -> Daten_einlesen
  data: int8x_1 input size=8; int8x_2 input size=8; int16x_bin output size=16 =0

== stateflow chart Gesamtsystem/Nexonar-System/Nexonar-Positionsbestimmung/Chart8 ==
  state wert_erkannt
    entry:
    values_out1[0] = in_data[0];
    values_out1[1] = in_data[1];
    values_out1[2] = in_data[2];
    values_out1[3] = in_data[3];
    values_out1[4] = in_data[4];
    values_out1[5] = in_data[5];
    values_out1[6] = in_data[6];
    values_out1[7] = in_data[7];
    values_out1[8] = in_data[8];
    values_out1[9] = in_data[9];
    values_out1[10] = in_data[10];
    values_out1[11] = in_data[11];
    values_out1[12] = in_data[12];
    values_out1[13] = in_data[13];
    values_out1[14] = in_data[14];
    values_out1[15] = in_data[15];
    values_out1[16] = in_data[16];
    values_out1[17] = in_data[17];
    values_out1[18] = in_data[18];
    values_out1[19] = in_data[19];
  state init
    entry: values_out1[0] = 0;
    values_out1[1] = 0;
    values_out1[2] = 0;
    values_out1[3] = 0;
    values_out1[4] = 0;
    values_out1[5] = 0;
    values_out1[6] = 0;
    values_out1[7] = 0;
    values_out1[8] = 0;
    values_out1[9] = 0;
    values_out1[10] = 0;
    values_out1[11] = 0;
    values_out1[12] = 0;
    values_out1[13] = 0;
    values_out1[14] = 0;
    values_out1[15] = 0;
    values_out1[16] = 0;
    values_out1[17] = 0;
    values_out1[18] = 0;
    values_out1[19] = 0;
  state Anfang_found_Schritt_uebertragen_weglassen_performance
    entry: x_found = x_found +1;
  state x5_valid_data_found1
    entry: valid_values1 = values_out1[search+1];
    valid_values2 = values_out1[search+2];
    valid_values3 = values_out1[search+3];
    valid_values4 = values_out1[search+4];
    valid_values5 = values_out1[search+5];
    valid_values6 = values_out1[search+6];
    valid_values7 = values_out1[search+7];
    valid_values8 = values_out1[search+8];
    zaehler = zaehler +1;
  state wert_erkannt2
    entry:
    search = 0;
    counter = counter + 1;
  state x1_search1
    entry: search = search + 1;
  x5_valid_data_found1 -> wert_erkannt
  (default) -> init
  x1_search1 -> wert_erkannt [order 3]
  init -> wert_erkannt
  Anfang_found_Schritt_uebertragen_weglassen_performance -> x5_valid_data_found1 [order 1] : [((values_out1[search]+values_out1[search+1]+values_out1[search+2]+values_out1[search+3]+values_out1[search+4]+values_out1[search+5]+values_out1[search+6]+values_out1[search+7]+values_out1[search+8])) == values_out1[search+9]]
  Anfang_found_Schritt_uebertragen_weglassen_performance -> x5_valid_data_found1 [order 2] : [((values_out1[search]+values_out1[search+1]+values_out1[search+2]+values_out1[search+3]+values_out1[search+4]+values_out1[search+5]+values_out1[search+6]+values_out1[search+7]+values_out1[search+8])-(256)) == values_out1[search+9]]
  wert_erkannt -> wert_erkannt2
  Anfang_found_Schritt_uebertragen_weglassen_performance -> x5_valid_data_found1 [order 3] : [((values_out1[search]+values_out1[search+1]+values_out1[search+2]+values_out1[search+3]+values_out1[search+4]+values_out1[search+5]+values_out1[search+6]+values_out1[search+7]+values_out1[search+8])-(512)) == values_out1[search+9]]
  Anfang_found_Schritt_uebertragen_weglassen_performance -> x5_valid_data_found1 [order 7] : [((values_out1[search]+values_out1[search+1]+values_out1[search+2]+values_out1[search+3]+values_out1[search+4]+values_out1[search+5]+values_out1[search+6]+values_out1[search+7]+values_out1[search+8])-(768)) == values_out1[search+9]]
  Anfang_found_Schritt_uebertragen_weglassen_performance -> x5_valid_data_found1 [order 6] : [((values_out1[search]+values_out1[search+1]+values_out1[search+2]+values_out1[search+3]+values_out1[search+4]+values_out1[search+5]+values_out1[search+6]+values_out1[search+7]+values_out1[search+8])-(1024)) == values_out1[search+9]]
  Anfang_found_Schritt_uebertragen_weglassen_performance -> x5_valid_data_found1 [order 5] : [((values_out1[search]+values_out1[search+1]+values_out1[search+2]+values_out1[search+3]+values_out1[search+4]+values_out1[search+5]+values_out1[search+6]+values_out1[search+7]+values_out1[search+8])-(1280)) == values_out1[search+9]]
  Anfang_found_Schritt_uebertragen_weglassen_performance -> x5_valid_data_found1 [order 4] : [((values_out1[search]+values_out1[search+1]+values_out1[search+2]+values_out1[search+3]+values_out1[search+4]+values_out1[search+5]+values_out1[search+6]+values_out1[search+7]+values_out1[search+8])-(1536)) == values_out1[search+9]]
  Anfang_found_Schritt_uebertragen_weglassen_performance -> x5_valid_data_found1 [order 8] : [((values_out1[search]+values_out1[search+1]+values_out1[search+2]+values_out1[search+3]+values_out1[search+4]+values_out1[search+5]+values_out1[search+6]+values_out1[search+7]+values_out1[search+8])-(1792)) == values_out1[search+9]]
  Anfang_found_Schritt_uebertragen_weglassen_performance -> x5_valid_data_found1 [order 10] : [((values_out1[search]+values_out1[search+1]+values_out1[search+2]+values_out1[search+3]+values_out1[search+4]+values_out1[search+5]+values_out1[search+6]+values_out1[search+7]+values_out1[search+8])-(2048)) == values_out1[search+9]]
  Anfang_found_Schritt_uebertragen_weglassen_performance -> x1_search1 [order 9]
  wert_erkannt2 -> Anfang_found_Schritt_uebertragen_weglassen_performance [order 1] : [values_out1[search] == 88]
  x1_search1 -> Anfang_found_Schritt_uebertragen_weglassen_performance [order 1] : [values_out1[search] == 88]
  wert_erkannt2 -> x1_search1 [order 2]
  x1_search1 -> x1_search1 [order 2] : [search < 19]
  data: in_data input size=20; values_out1 local int16 size=20; zaehler local int32 =0; search local int16; valid_values1 output int16 size=1; valid_values2 output int16 size=1; valid_values3 output int16 size=1; valid_values4 output int16 size=1; valid_values5 output int16 size=1; valid_values6 output int16 size=1; valid_values7 output int16 size=1; valid_values8 output int16 size=1; counter local int32 =0; x_found local int32 =0

== matlab function Gesamtsystem/Nexonar-System/Navigationssystem [Einstellungen moeglich]/Positionsregelungssystem (Soll-Ist-Abgleich & PWM-Auswertung)/Betrag pwm_x ==
  settings: updateMethod=DISCRETE  sampleTime=0.01
  data: x_diff_abs input; pwm_x output; Zielradius input
function pwm_x = fcn( x_diff_abs, Zielradius)

if Zielradius < x_diff_abs && x_diff_abs < 60 + Zielradius
    pwm_x = 60;
elseif x_diff_abs <= Zielradius
    pwm_x = 0;
elseif x_diff_abs >= 100 + Zielradius
    pwm_x = 100;
else
    pwm_x = x_diff_abs;
end

== matlab function Gesamtsystem/Nexonar-System/Navigationssystem [Einstellungen moeglich]/Positionsregelungssystem (Soll-Ist-Abgleich & PWM-Auswertung)/Betrag pwm_y ==
  settings: updateMethod=DISCRETE  sampleTime=0.01
  data: Zielradius input; y_diff_abs input; pwm_y output
function pwm_y = fcn(Zielradius, y_diff_abs)

if Zielradius < y_diff_abs && y_diff_abs < 60 + Zielradius
    pwm_y = 60;
elseif y_diff_abs <= Zielradius
    pwm_y = 0;
elseif y_diff_abs >= 100 + Zielradius
    pwm_y = 100;
else
    pwm_y = y_diff_abs;
end

== matlab function Gesamtsystem/Nexonar-System/Nexonar-Positionsbestimmung/I2C Reset (behebt Stabilitätsprobleme der I2C-Verbindung)/I2C Reset/I2C Reset ==
function fcn()
%#codegen

coder.ceval( 'reset_i2c' );

== matlab function Gesamtsystem/Nexonar-System/Nexonar-Positionsbestimmung/I2C Reset (behebt Stabilitätsprobleme der I2C-Verbindung)/I2C Reinitialisierung/I2C Reinitialisierung ==
function fcn()
%#codegen

coder.ceval( 'init_i2c' );

== stateflow chart Gesamtsystem/Subsystem/Chart6 ==
  state closeKlappe
    gatePWM = 100;
    gateDirection = 0;
  state close
    gateDirection = 0
  state wait
    gateDirection = 0
    gatePWM = 60;
    movingCube = 0
  state open
    gateDirection = 1;
    gatePWM = 100
    movingCube = 1
  state CloseRegular
    gatePWM = 100;
    gateDirection = 0
  closeKlappe -> wait : [after(1,sec)]
  wait -> closeKlappe [order 2] : [signal == (-1)]
  (default) -> wait
  wait -> open [order 1] : [signal == 1]
  open -> close : [after(0.5,sec)]
  close -> wait : [after(0.4, sec)]
  data: signal input; gatePWM output; gateDirection output; movingCube output single

== stateflow chart Gesamtsystem/Subsystem/Chart7 ==
  state startPosition
    entry: angle = 0;
  state firstEntry
    entry: angle = 300;
    signal = -1;
  note: StartWinkel, da Schieber nicht in Mitte stehen darf am Anfang. 5 Sekunden Zeit um das Bord einzuschalten
  state closeKlappe
    signal = 0;
  state betterRightPosition
    angle = 220;
  state waitForCube
  state goToZero
    angle = 0;
    movingCube = 1
  state betterLeftPosition
    angle = -170;
  state closeGate
    signal = 0
  state wait
  state openGate
    signal = 1
    movingCube = 0
  state goToMagacin
    entry: angle = magacin;
  (default) -> startPosition
  startPosition -> firstEntry : [switchA > 0]
  firstEntry -> closeKlappe : [after(0.7,sec)]
  closeKlappe -> waitForCube : [after(2.3,sec)]
  betterRightPosition -> waitForCube
  waitForCube -> betterRightPosition [order 1] : [angle == 85]
  waitForCube -> goToZero [order 3] : [magacin ~= -1]
  betterLeftPosition -> waitForCube
  goToZero -> wait : [(inputAngle > -2) && (inputAngle < 2)]
  waitForCube -> betterLeftPosition [order 2] : [angle == -40]
  closeGate -> waitForCube : [cubeFinished == 0]
  openGate -> closeGate : [after(0.5, sec)]
  wait -> goToMagacin : [after(0.4, sec)]
  goToMagacin -> openGate : [(inputAngle > (angle - 2)) && (inputAngle < (angle + 2))]
  data: inputAngle input; magacin input; angle output; signal output; movingCube output single; cubeFinished input; switchA input

== stateflow chart Gesamtsystem/Subsystem/Chart8 ==
  state end
    gatePWM = 100;
    gateDirection = 1;
    panzerMotor = 0;
  state Stillstand
    gatePWM = 0;
  state Lampe
    lampe = 1;
  state entry
    tasterCounter = 0;
    panzerMotor = 0;
    lampe = 0;
  state wait1
    gatePWM = 0;
  state open
    entry: tasterCounter = tasterCounter + 1;
    gatePWM = 100
    gateDirection = 0;
    panzerMotor = 1;
  state wait
    gatePWM = 0;
    gateDirection = 0;
  (default) -> entry
  end -> Stillstand : [after(0.5,sec)]
  Stillstand -> Lampe : [after(1,sec)]
  wait -> end [order 1] : [(signal > 0) && (tasterCounter >= 2)]
  entry -> wait
  open -> wait1 : [after(0.5,sec)]
  wait -> open [order 2] : [signal > 0 && tasterCounter == 0]
  wait1 -> wait : [after(2,sec)]
  wait -> wait [order 3] : [(signal > 0) && (tasterCounter == 1)]{tasterCounter = 2;}
  data: signal input; gatePWM output; gateDirection output; tasterCounter local; panzerMotor output; lampe output

== matlab function Gesamtsystem/Subsystem/P-Regler mit Output2/P-Regler mit Regelfehler Begrenzung Initial: k = 0.1, limiit = +//- 100 Sampletime 0.01/Betrag ==
  settings: updateMethod=DISCRETE  sampleTime=0.01
  data: u input; y output
function y = fcn( u )

if 0.5 < u && u < 60
    y = 60;
elseif u <= 0.5
    y = 0;
elseif u >= 100
    y = 100;
else
    y = abs(u);
end

== matlab function Gesamtsystem/Subsystem/P-Regler mit Output2/P-Regler mit Regelfehler Begrenzung Initial: k = 0.1, limiit = +//- 100 Sampletime 0.01/Richtung ==
  settings: updateMethod=DISCRETE  sampleTime=0.01
  data: u input; y output
function y = fcn( u )

if u > 0
    y = 1;
else
    y = 0;
end

== stateflow chart Gesamtsystem/Subsystem/Sortieralgorithmus2 ==
  state setupVariable
    magacin0 = 0;
    magacin1 = 0;
    magacin2 = 0;
    magacin3 = 0;
    magacin4 = 0;
    magacin5 = 0;
    magacin6 = 0;
    magacin0_LastCube = 0;
    magacin1_LastCube = 0;
    magacin2_LastCube = 0;
    magacin3_LastCube = 0;
    magacin4_LastCube = 0;
    magacin5_LastCube = 0;
    magacin6_LastCube = 0;
    magacin = -1;
    cubeCounter = 0
    signal = 0;
  state cubeLoaded
    magacin = -1
  state photoelectricBarrierActivated
  state BlueCube
    entry: magacin = findPlaceForBlue();
  state RedCube
    entry: magacin = findPlaceForRed();
  state Black
    magacin = 6;
  state DetectedCube
    entry: cubeCounter = cubeCounter + 1;
  setupVariable -> cubeLoaded : [switchA > 0]
  (default) -> setupVariable
  DetectedCube -> cubeLoaded : [movingCube == 0]
  cubeLoaded -> photoelectricBarrierActivated : [(colour < 700) || (colour > 1500)]
  photoelectricBarrierActivated -> BlueCube [order 3] : [((colour >= 1000) && (colour <= 2150)) ]
  photoelectricBarrierActivated -> RedCube [order 2] : [(colour < 1000)]
  photoelectricBarrierActivated -> Black [order 1] : [(colour > 2150) ]
  Black -> DetectedCube
  RedCube -> DetectedCube
  BlueCube -> DetectedCube
  data: magacinOut function_output; magacinOut function_output; colour input; magacin6 local; magacin0_LastCube local; magacin3_LastCube local; magacin2_LastCube local; magacin5_LastCube local; magacin1_LastCube local; magacin6_LastCube local; magacin4_LastCube local; magacin output; magacin0 local; magacin1 local; magacin2 local; magacin3 local; magacin4 local; magacin5 local; movingCube input; cubeCounter local; signal output; switchA input
  function magacinOut  = findPlaceForRed:
    | function magacinOut  = findPlaceForRed
    | 
    | if((magacin1 == 0) || ((magacin1_LastCube == 1)&& (magacin1 < 5)))
    |             magacinOut = 1;
    |             magacin1 = magacin1 + 1;
    |             magacin1_LastCube = 2;
    |             position = magacin1;
    | elseif (((magacin2_LastCube == 1) && (magacin2 < 5)))
    |             magacinOut = 2;
    |             magacin2 = magacin2 + 1; 
    |             magacin2_LastCube = 2;
    |             position = magacin2;
    | elseif (magacin0 ~= 5)
    |             magacinOut = 0;
    |             magacin0 = magacin0 + 1;
    |             magacin0_LastCube = 2;
    |             position = magacin0;
    | else
    |         if (magacin3 ~= 5)
    |                 magacinOut = 3;
    |                 magacin3 = magacin3 + 1; 
    |                 magacin3_LastCube = 2;
    |                 position = magacin3;
    |         elseif ((magacin1 <= magacin4) && (magacin1 ~= 5))
    |                 magacinOut = 1;
    |                 magacin1 = magacin1 + 1; 
    |                 magacin1_LastCube = 2;
    |                 position = magacin1;
    |         elseif (magacin1 > magacin4)
    |                 magacinOut = 4;
    |                 magacin4 = magacin4 + 1;
    |                 magacin4_lastCube = 2;
    |                 position = magacin4;
    |         elseif ((magacin2 <= magacin5) && (magacin2 ~= 5))
    |                 magacinOut = 2;
    |                 magacin2 = magacin2 + 1;
    |                 magacin2_LastCube = 2;
    |                 position = magacin2;
    |         elseif (magacin2 > magacin5)
    |             
    |                 magacinOut = 5;
    |                 magacin5 = magacin5 + 1;
    |                 magacin5_LastCube = 2;
    |                 position = magacin5;
    |         else
    |                 magacinOut = -1;
    |         end            
    | end
  function magacinOut  = findPlaceForBlue:
    | function magacinOut  = findPlaceForBlue
    | 
    | %1 ist Code for Blue, 2 is Code for Red, 3 is Code for Black, 0 is empty
    | if(magacin0 == 4)  
    |             magacinOut = 0;
    |             magacin0 = (magacin0 + 1);
    |             magacin0_LastCube = 1;
    |             position = magacin0;
    | elseif ((magacin2 == 0) || (magacin2_LastCube == 2 && magacin2 < 5))
    |             magacinOut = 2;
    |             magacin2 = magacin2 + 1; 
    |             magacin2_LastCube = 1;
    |             position = magacin2;
    | elseif ((magacin1_LastCube == 2) && (magacin1 < 5))
    |             magacinOut = 1;
    |             magacin1 = magacin1 + 1;
    |             magacin1_LastCube = 1;
    |             position = magacin1;
    | elseif (magacin3 < 5)
    |             magacinOut = 3;
    |             magacin3 = (magacin3 + 1);
    |             position = magacin3;
    | elseif (magacin4 < 5)
    |             magacinOut = 4;
    |             magacin4 = (magacin4 + 1);
    |             position = magacin4;
    | elseif (magacin5 < 5)
    |             magacinOut = 5;
    |             magacin5 = (magacin5 + 1);
    |             position = magacin5;
    | else
    |             magacinOut = -1
    | end

== matlab function Gesamtsystem/Subsystem/getAngle2/Messung des absoluten Winkels - Auswertung der Encodersignale/MATLAB Function1 ==
  data: u input; y output; yalt input
function y = fcn(u, yalt)

y = yalt + u;
